simulink model "simula_ajuste_siso"  (R2018a)
settings: Solver=VariableStepAuto  StartTime=0.0  StopTime=Tsim  RelTol=1e-3
values from neighbouring files (symbols this model uses):
  delta = [1 -1]    [ajuste_mimo.m]    (also in ajuste_siso.m)
  Ke = Ku * E    [ajuste_mimo.m]    (also in ajuste_siso.m = K(1,:) * E)
  Kf = Ku * F    [ajuste_mimo.m]    (also in ajuste_siso.m = K(1,:) * F)
  Kr = Kr + Ku(1:nin,nin*i-1:nin*i)    [ajuste_mimo.m]
  Ts = 0.03    [ajuste_mimo.m]    (also in ajuste_siso.m = 0.1)
  Tsim = 8    [ajuste_mimo.m]    (also in ajuste_siso.m = 20)
libraries: cstblocks x5
settings Model: Creator=aluno-4  LastModifiedBy=marcus

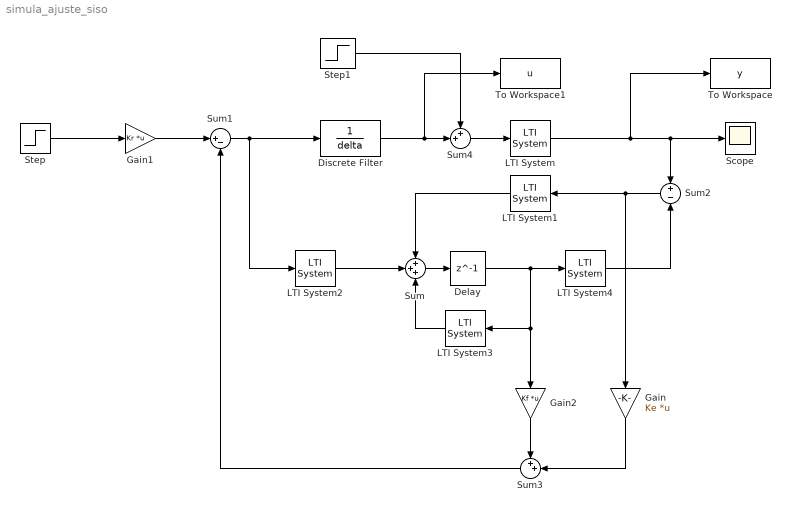
== system simula_ajuste_siso ==
  Delay : Delay  DelayLength=1
  Discrete Filter : DiscreteFilter  Numerator=1  Denominator=delta  SampleTime=Ts
  Gain : Gain  Gain=Ke  Multiplication=Matrix(K*u)
  Gain1 : Gain  Gain=Kr  Multiplication=Matrix(K*u)
  Gain2 : Gain  Gain=Kf  Multiplication=Matrix(K*u)
  LTI System : cstblocks/LTI System  sys=P  IC=[]
  LTI System1 : cstblocks/LTI System  sys=D  IC=[]
  LTI System2 : cstblocks/LTI System  sys=B  IC=[]
  LTI System3 : cstblocks/LTI System  sys=A  IC=[]
  LTI System4 : cstblocks/LTI System  sys=H  IC=[]
  Scope : Scope
  Step : Step  Time=0  SampleTime=0
  Step1 : Step  Time=Tsim/2  SampleTime=0
  Sum : Sum  Inputs=+++
  Sum1 : Sum  Inputs=|+-
  Sum2 : Sum  Inputs=+-
  Sum3 : Sum  Inputs=++|
  Sum4 : Sum  Inputs=++|
  To Workspace : ToWorkspace  VariableName=y  SaveFormat=Timeseries  SampleTime=-1
  To Workspace1 : ToWorkspace  VariableName=u  SaveFormat=Timeseries  SampleTime=Ts
  wires:
  Discrete Filter/1 -> To Workspace1/1, Sum4/2
  Sum1/1 -> LTI System2/1, Discrete Filter/1
  Step/1 -> Gain1/1
  LTI System2/1 -> Sum/2
  LTI System1/1 -> Sum/1
  Sum/1 -> Delay/1
  Delay/1 -> LTI System4/1, Gain2/1, LTI System3/1
  LTI System3/1 -> Sum/3
  LTI System/1 -> Scope/1, Sum2/1, To Workspace/1
  LTI System4/1 -> Sum2/2
  Sum2/1 -> LTI System1/1, Gain/1
  Gain/1 -> Sum3/2
  Gain2/1 -> Sum3/1
  Sum3/1 -> Sum1/2
  Gain1/1 -> Sum1/1
  Step1/1 -> Sum4/1
  Sum4/1 -> LTI System/1
